simulink model "Part2_LQ"  (R2021a)
settings: Solver=ode45  StartTime=0.0  StopTime=24  MaxStep=0.01  RelTol=1e-3  EnableMultiTasking=on
values from neighbouring files (symbols this model uses):
  A = [0 1; -K/m -D/m]    [Part1.m]    (also in Part2.m = [zeros(2) eye(2))
  B = [0 ; 1]    [Part1.m]    (also in Part2.m = [zeros(2,1))
  Bp = [0 ; 1 ]    [Part1.m]    (also in Part2.m = [zeros(2,1))
  C = [1 0]    [Part1.m]    (also in Part2.m = [1 0 0 0])
  K_LQ = lqr(sys, Q, r^2)    [Part2.m]
  seisme =     [seisme.mat]
settings Model: Creator=Tebbani  LastModifiedBy=Sihem Tebbani
settings SolverCC: AlgebraicLoopSolver=TrustRegion
settings DataIOCC: LimitDataPoints=on  SaveFormat=Array  ReturnWorkspaceOutputs=off
settings OptimizationCC: LifeSpan=inf
settings DebuggingCC: SolverPrmCheckMsg=warning  SFUnexpectedBacktrackingDiag=warning  SFNoUnconditionalDefaultTransitionDiag=warning  SFExecutionAtInitializationDiag=none  SFMachineParentedDataDiag=warning  ArithmeticOperatorsInVariantConditions=warning
settings HardwareCC: ProdBitPerPointer=32  ProdBitPerSizeT=32  ProdBitPerPtrDiffT=32  ProdLargestAtomicFloat=None  ProdIntDivRoundTo=Undefined  ProdEndianess=Unspecified  ProdWordSize=32  ProdHWDeviceType=32-bit Generic
settings ModelReferenceCC: PropagateSignalLabelsOutOfModel=off
settings SFSimCC: SimUseLocalCustomCode=off  CustomCodeUndefinedFunction=UseInterfaceOnly
settings RTWCC: RTWUseLocalCustomCode=off
settings CodeAppCC: StateflowObjectComments=on
settings GRTTargetCC: TargetLangStandard=C89/C90 (ANSI)
settings ConfigComp: CovMetricSettings=dw  CovSaveCumulativeToWorkspaceVar=on  CovSaveSingleToWorkspaceVar=on  CovExternalEMLEnable=off  CovSFcnEnable=off

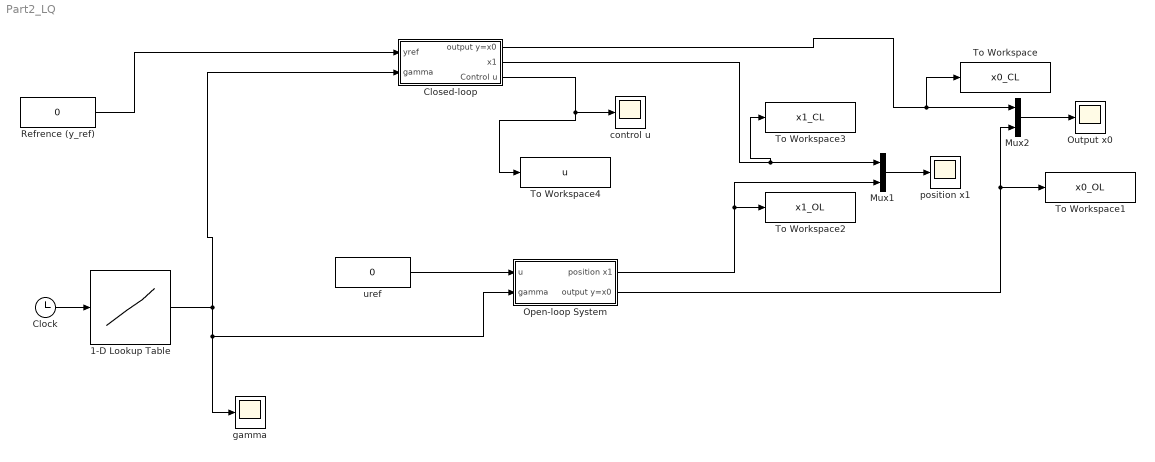
== system Part2_LQ ==
  1-D Lookup Table : Lookup_n-D  NumberOfTableDimensions=1  BreakpointsForDimension1=seisme.time  BeginIndexSearchUsingPreviousIndexResult=on  Table=seisme.signals.values  RemoveProtectionInput=on  InternalRulePriority=Speed  RndMeth=Simplest  InputSameDT=on
  Clock : Clock
  Closed-loop : Subsystem
  Mux1 : Mux  Inputs=2
  Mux2 : Mux  Inputs=2
  Open-loop System : Subsystem
  "Output x0 " : Scope
  Refrence (y_ref) : Constant  Value=0
  To Workspace : ToWorkspace  VariableName=x0_CL  SaveFormat=Structure With Time  SampleTime=-1
  To Workspace1 : ToWorkspace  VariableName=x0_OL  SaveFormat=Structure With Time  SampleTime=-1
  To Workspace2 : ToWorkspace  VariableName=x1_OL  SaveFormat=Structure With Time  SampleTime=-1
  To Workspace3 : ToWorkspace  VariableName=x1_CL  SaveFormat=Structure With Time  SampleTime=-1
  To Workspace4 : ToWorkspace  VariableName=u  SaveFormat=Structure With Time  SampleTime=-1
  control u : Scope
  gamma : Scope
  position x1 : Scope
  uref : Constant  Value=0
  wires:
  Mux2/1 -> "Output x0 "/1
  Refrence (y_ref)/1 -> Closed-loop/1(yref)
  Clock/1 -> 1-D Lookup Table/1
  1-D Lookup Table/1 -> Closed-loop/2(gamma), gamma/1, Open-loop System/2(gamma)
  uref/1 -> Open-loop System/1(u)
  Closed-loop/1(output y=x0) -> To Workspace/1, Mux2/1
  Closed-loop/3(Control u) -> To Workspace4/1, control u/1
  Closed-loop/2(x1) -> To Workspace3/1, Mux1/1
  Mux1/1 -> position x1/1
  Open-loop System/1(position x1) -> To Workspace2/1, Mux1/2
  Open-loop System/2(output y=x0) -> To Workspace1/1, Mux2/2

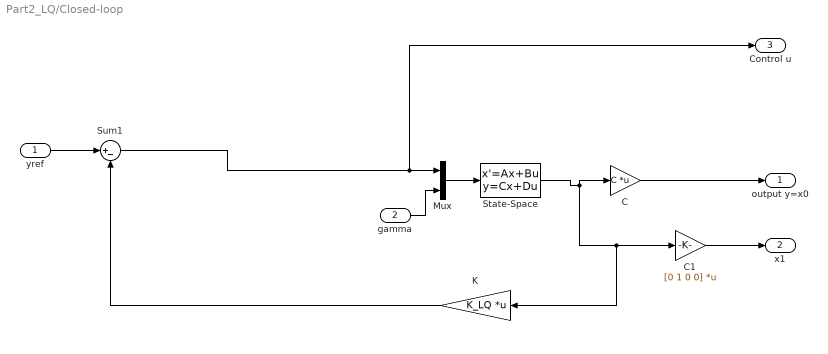
== system Part2_LQ/Closed-loop ==
  yref : Inport
  gamma : Inport  Port=2
  C : Gain  Gain=C  Multiplication=Matrix(K*u) (u vector)
  C1 : Gain  Gain=[0 1 0 0]  Multiplication=Matrix(K*u) (u vector)
  K : Gain  Gain=K_LQ  Multiplication=Matrix(K*u) (u vector)
  Mux : Mux  Inputs=2
  State-Space : StateSpace  A=A  B=[B Bp]  C=eye(4)  D=zeros(4,2)  InitialCondition=0
  Sum1 : Sum  Inputs=|+-
  output y=x0 : Outport
  x1 : Outport  Port=2
  Control u : Outport  Port=3
  wires:
  C/1 -> output y=x0/1
  State-Space/1 -> C/1, K/1, C1/1
  gamma/1 -> Mux/2
  Mux/1 -> State-Space/1
  yref/1 -> Sum1/1
  K/1 -> Sum1/2
  C1/1 -> x1/1
  Sum1/1 -> Control u/1, Mux/1

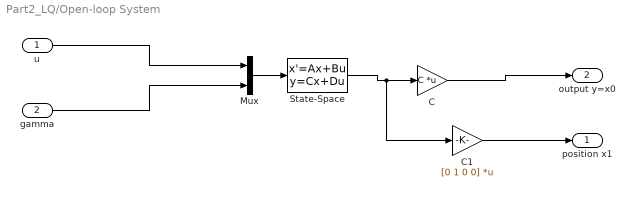
== system Part2_LQ/Open-loop System ==
  u : Inport
  gamma : Inport  Port=2
  C : Gain  Gain=C  Multiplication=Matrix(K*u) (u vector)
  C1 : Gain  Gain=[0 1 0 0]  Multiplication=Matrix(K*u) (u vector)
  Mux : Mux  Inputs=2
  State-Space : StateSpace  A=A  B=[B Bp]  C=eye(4)  D=zeros(4,2)  InitialCondition=0
  position x1 : Outport
  output y=x0 : Outport  Port=2
  wires:
  Mux/1 -> State-Space/1
  gamma/1 -> Mux/2
  u/1 -> Mux/1
  State-Space/1 -> C1/1, C/1
  C/1 -> output y=x0/1
  C1/1 -> position x1/1
